simulink model "space-state-marotage"  (R2014b)
settings: Solver=ode14x  StartTime=0.0  StopTime=inf  FixedStep=0.1  RelTol=1e-3
undefined symbols (not defined in the file or in its folder): A, B, C, IsPositionTracked, IsSkeletonTracked, JointDepthIndices, JointImageIndices, JointTrackingState, JointWorldCoordinates, K, L, none, PositionDepthIndices, PositionImageIndices, PositionWorldCoordinates, SegmentationData, SkeletonTrackingID, videoinput
libraries: simulink x6, arduino_io_lib x2, visionsinks x2, visionstatistics x1, visiontextngfix x1, imaqlib x1, visiongeotforms x1
settings Model: Creator=mtsou_000  LastModifiedBy=mtsou_000

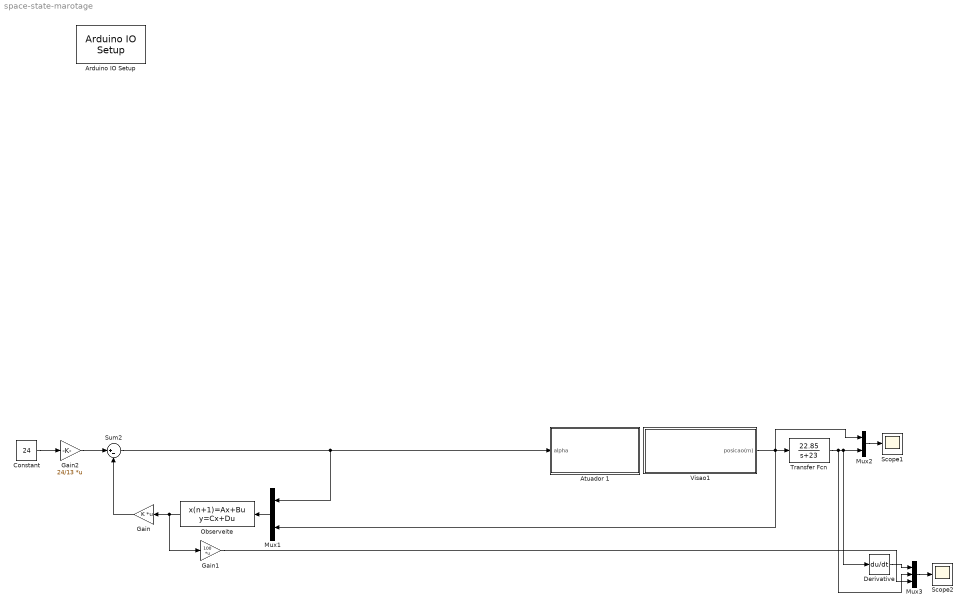
== system space-state-marotage ==
  Arduino IO Setup : arduino_io_lib/Arduino IO Setup  Priority=3  arduinoVar=Temporary arduino variable: Arduino1  workspaceVarName=a  comPort=COM8
  Atuador 1 : Subsystem
  Constant : Constant  Value=24
  Derivative : Derivative
  Gain : Gain  Gain=K  Multiplication=Matrix(K*u)
  Gain1 : Gain  Gain=100  Multiplication=Matrix(K*u)
  Gain2 : Gain  Gain=24/13  Multiplication=Matrix(K*u)
  Mux1 : Mux  Inputs=2
  Mux2 : Mux  Inputs=3
  Mux3 : Mux  Inputs=3
  Observeite : DiscreteStateSpace  A=A-L*C  B=[B L]  C=eye(2)  D=zeros(2)  SampleTime=0.1
  Scope1 : Scope
      settings: TimeRange=10  YMin=0  YMax=35  SaveName=ScopeData3
  Scope2 : Scope
      settings: TimeRange=10  YMin=-20  YMax=30
  Sum2 : Sum  Inputs=|+-
  Transfer Fcn : TransferFcn  Numerator=[22.85]  Denominator=[1 23]
  Visao1 : Subsystem
  wires:
  Observeite/1 -> Gain1/1, Gain/1
  Mux1/1 -> Observeite/1
  Mux2/1 -> Scope1/1
  Visao1/1(posicao(m)) -> Mux2/1, Mux1/2, Transfer Fcn/1
  Gain/1 -> Sum2/2
  Constant/1 -> Gain2/1
  Sum2/1 -> Atuador 1/1(alpha), Mux1/1
  Gain2/1 -> Sum2/1
  Transfer Fcn/1 -> Mux3/2, Derivative/1, Mux2/3
  Mux3/1 -> Scope2/1
  Derivative/1 -> Mux3/1
  Gain1/1 -> Mux3/3

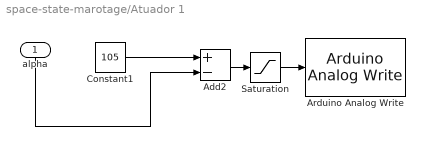
== system space-state-marotage/Atuador 1 ==
  alpha : Inport
  Add2 : Sum  Inputs=+-
  Arduino Analog Write : arduino_io_lib/Arduino Analog Write  arduinoVar=Temporary arduino variable: Arduino1  arduinoPin=3  T=0.1
  Constant1 : Constant  Value=105
  Saturation : Saturate  UpperLimit=120  LowerLimit=60
  wires:
  Add2/1 -> Saturation/1
  alpha/1 -> Add2/2
  Saturation/1 -> Arduino Analog Write/1
  Constant1/1 -> Add2/1

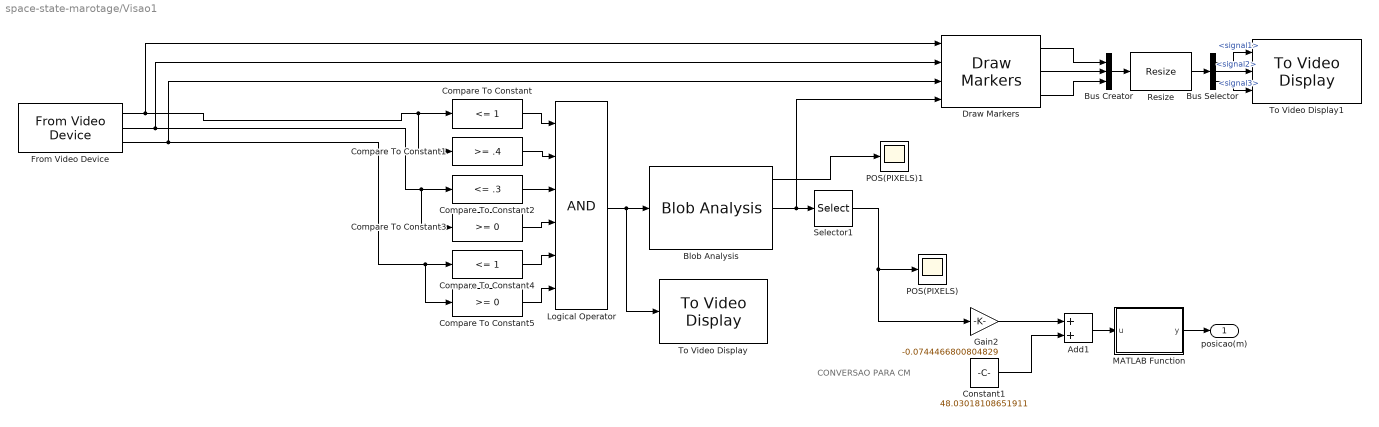
== system space-state-marotage/Visao1 ==
  note: CONVERSAO PARA CM
  Add1 : Sum
  Blob Analysis : visionstatistics/Blob Analysis  Tag=vipblks_row_conv  area=on  centroid=on  bBox=off  majorAxis=off  minorAxis=off  angle=off  eccentricity=off  equivDiameterSq=on  extent=off  perimeter=off  maxBlobs=1  warnIfNumBlobsExceeded=off  isCount=off  useMinArea=on  minArea=400  useMaxArea=off  maxArea=2200  excludeBorderBlob=off  outDT=double  isOutVarDim=off  isFill=on  fillValues=-1  conn=8  isLabel=off  outputMode=Binary point scaling  outputWordLength=32  outputFracLength=16  firstCoeffMode=Binary point scaling  firstCoeffWordLength=16  firstCoeffFracLength=14  secondCoeffMode=Binary point scaling  secondCoeffWordLength=32  secondCoeffFracLength=16  accumMode=Binary point scaling  accumWordLength=32  accumFracLength=0  prodOutputMode=Binary point scaling  prodOutputWordLength=32  prodOutputFracLength=16  roundingMode=Floor  overflowMode=off
  Bus Creator : BusCreator  Inputs=3
  Bus Selector : BusSelector
  Compare To Constant : simulink/Logic and Bit Operations/Compare To Constant  relop=<=  const=1  OutDataTypeStr=boolean
  Compare To Constant1 : simulink/Logic and Bit Operations/Compare To Constant  relop=>=  const=.4  OutDataTypeStr=boolean
  Compare To Constant2 : simulink/Logic and Bit Operations/Compare To Constant  relop=<=  const=.3  OutDataTypeStr=boolean
  Compare To Constant3 : simulink/Logic and Bit Operations/Compare To Constant  relop=>=  const=0  OutDataTypeStr=boolean
  Compare To Constant4 : simulink/Logic and Bit Operations/Compare To Constant  relop=<=  const=1  OutDataTypeStr=boolean
  Compare To Constant5 : simulink/Logic and Bit Operations/Compare To Constant  relop=>=  const=0  OutDataTypeStr=boolean
  Constant1 : Constant  Value=48.03018108651911
  Draw Markers : visiontextngfix/Draw Markers  shape=Circle  size=28  fill=on  fillClrSource=Specify via dialog  display=White  intensity=200  color=[200 255 100]  opacity=.5  viewport=Entire image  antialiasing=off  inType=Obsolete  imagePorts=Separate color signals  prodOutputMode=Binary point scaling  prodOutputWordLength=32  prodOutputFracLength=14  memoryMode=Specify word length  memoryWordLength=16  memoryFracLength=14  roundingMode=Floor  overflowMode=off
  From Video Device : imaqlib/From Video Device  DeviceMenu=winvideo 1 (Lenovo EasyCamera)  Device=winvideo 2 (Webcam 1200)  ObjConstructor=videoinput('winvideo', 2)  VideoFormatMenu=MJPG_1280x720  VideoFormat=RGB24_640x480  VideoSource=input1  ROIPosition=[0 0 480 640]  EnableHWTrigger=off  TriggerConfiguration=none/none  SampleTime=0.1  OutputPortsMode=Separate color signals  DataType=single  CanDoHWTrigger=no  ReturnedColorSpace=rgb  BlockHandle=1921.0006  ROIWidth=640  ROIHeight=480  ROIColumn=0  ROIRow=0  EngXMLPath=C:\Program Files\MATLAB\R2014b\toolbox\imaq\imaq\private  DevXMLPath=C:\MATLAB\SupportPackages\R2014b\osgenericvideointerface\toolbox\imaq\supportpackages\genericvideo\adaptor\win64  EngLibPath=C:\Program Files\MATLAB\R2014b\toolbox\imaq\imaqblks\imaqmex\win64  ColorSpace=rgb  BayerSensorAlignment=grbg  AllMetadata=IsPositionTracked;IsSkeletonTracked;JointDepthIndices;JointImageIndices;JointTrackingState;JointWorldCoordinates;PositionDepthIndices;PositionImageIndices;PositionWorldCoordinates;SegmentationData;SkeletonTrackingID
  Gain2 : Gain  Gain=-0.0744466800804829
  Logical Operator : Logic  Inputs=6  AllPortsSameDT=off  OutDataTypeStr=boolean
  MATLAB Function : MATLAB Function  TreatAsAtomicUnit=on
  POS(PIXELS) : Scope
      settings: YMin=-2  YMax=0
  POS(PIXELS)1 : Scope
      settings: YMin=-500  YMax=2500  SaveName=ScopeData2
  Resize : visiongeotforms/Resize  specify=Number of output rows and columns  rfactor=[200 150]  outCols=25  outRows=25  outRowsCols=[300 400]  interp_method=Bilinear  antialias=on  useROI=off  roiFlag=off  prodOutputMode=Binary point scaling  prodOutputWordLength=32  prodOutputFracLength=10  roundingMode=Nearest  overflowMode=on
  Selector1 : Selector  NumberOfDimensions=2  InputPortWidth=2  IndexOptions=Index vector (dialog),Index vector (dialog)  Indices=1,1  OutputSizes=1,1
  To Video Display : visionsinks/To Video Display  inputType=Obsolete  imagePorts=One multidimensional signal  OutputDevice=On-screen video monitor  fullScreen=off  videoWindowX=684  videoWindowY=-1  saveWindowSize=off  videoWindowWidth=640  videoWindowHeight=480  dataOrg=Column-major  openAtMdlStart=on  isWindowOpen=on  inputColorFormat=RGB
  To Video Display1 : visionsinks/To Video Display  inputType=Obsolete  imagePorts=Separate color signals  OutputDevice=On-screen video monitor  fullScreen=off  videoWindowX=813  videoWindowY=179  saveWindowSize=off  videoWindowWidth=400  videoWindowHeight=300  dataOrg=Column-major  openAtMdlStart=on  isWindowOpen=on  inputColorFormat=RGB
  posicao(m) : Outport
  wires:
  Compare To Constant5/1 -> Logical Operator/6
  From Video Device/3 -> Draw Markers/3, Compare To Constant5/1, Compare To Constant4/1
  Compare To Constant/1 -> Logical Operator/1
  Logical Operator/1 -> To Video Display/1, Blob Analysis/1
  Compare To Constant1/1 -> Logical Operator/2
  From Video Device/2 -> Draw Markers/2, Compare To Constant2/1, Compare To Constant3/1
  Compare To Constant2/1 -> Logical Operator/3
  Compare To Constant4/1 -> Logical Operator/5
  Compare To Constant3/1 -> Logical Operator/4
  From Video Device/1 -> Draw Markers/1, Compare To Constant/1, Compare To Constant1/1
  Blob Analysis/2 -> Selector1/1, Draw Markers/4
  Bus Creator/1 -> Resize/1
  Resize/1 -> Bus Selector/1
  Bus Selector/1 -> To Video Display1/1  "<signal1>"
  Bus Selector/2 -> To Video Display1/2  "<signal2>"
  Bus Selector/3 -> To Video Display1/3  "<signal3>"
  Draw Markers/2 -> Bus Creator/2
  Draw Markers/1 -> Bus Creator/1
  Draw Markers/3 -> Bus Creator/3
  Selector1/1 -> Gain2/1, POS(PIXELS)/1
  Gain2/1 -> Add1/1
  Constant1/1 -> Add1/2
  Add1/1 -> MATLAB Function/1(u)
  Blob Analysis/1 -> POS(PIXELS)1/1
  MATLAB Function/1(y) -> posicao(m)/1

== matlab function space-state-marotage/Visao1/MATLAB Function ==
  data: u input; y output
function y = fcn(u)

persistent float ua;

if (isempty(ua))
    ua = 20;
end

if (abs(u-ua)>25)
    u = ua;
end

ua = u;
y=u;
